simulink model "walkingRobotRL3D"  (R2020b)
settings: Solver=ode23t  StartTime=0.0  StopTime=Tf  RelTol=1e-2  EnableMultiTasking=on
PreLoadFcn:
  | robotParametersRL
undefined symbols (not defined in the file): agent, ankleD_pitch_jointMAX, ankleD_pitch_jointMIN, ankleD_roll_jointMAX, ankleD_roll_jointMIN, ankleI_pitch_jointMAX, ankleI_pitch_jointMIN, ankleI_roll_jointMAX, ankleI_roll_jointMIN, getSampleTime, height_plane, hipD_pitch_jointMAX, hipD_pitch_jointMIN, hipD_roll_jointMAX, hipD_roll_jointMIN, hipI_pitch_jointMAX, hipI_pitch_jointMIN, hipI_roll_jointMAX, hipI_roll_jointMIN, init_angs_L, init_angs_R, init_height, joint_damping, joint_limit_damping, joint_limit_stiffness, joint_stiffness, kneeD_jointMAX, kneeD_jointMIN, kneeI_jointMAX, kneeI_jointMIN, lower_leg_I0, lower_leg_length, lower_leg_mass, lower_leg_x, lower_leg_y, muscle_nominal_length, p10_ankleD_roll, plane_x, plane_y, regulator_type, tau, Tf, torso_height, torso_length, torso_offset_x, torso_offset_z, torso_width, torso_x, torso_y, torso_z, Ts, upper_leg_I0, upper_leg_length, upper_leg_mass, upper_leg_x, upper_leg_y, v10_ankleD_pitch, v10_ankleD_roll, v10_ankleI_pitch, v10_ankleI_roll ... (+41)
libraries: sm_lib x222, simulink x183, nesl_utility x130, walkingRobotUtils x69, rllib x2
(part 4 of 24)

== system walkingRobotRL3D/Calculate Reward3/Check correct behaviour of the muscles ==
  actions : Inport
  Add : Sum  Inputs=++++++++++
  Demux : Demux  Outputs=20
  Subsystem : Subsystem
  Subsystem1 : Subsystem
  Subsystem2 : Subsystem
  Subsystem3 : Subsystem
  Subsystem4 : Subsystem
  Subsystem5 : Subsystem
  Subsystem6 : Subsystem
  Subsystem7 : Subsystem
  Subsystem8 : Subsystem
  Subsystem9 : Subsystem
  Muscles checked : Outport
  wires:
  actions/1 -> Demux/1
  Demux/1 -> Subsystem/1(In1)
  Demux/2 -> Subsystem/2(In2)
  Subsystem/1(Out1) -> Add/1
  Demux/3 -> Subsystem1/1(In1)
  Demux/4 -> Subsystem1/2(In2)
  Subsystem1/1(Out1) -> Add/2
  Demux/7 -> Subsystem3/1(In1)
  Demux/8 -> Subsystem3/2(In2)
  Demux/9 -> Subsystem4/1(In1)
  Demux/10 -> Subsystem4/2(In2)
  Demux/11 -> Subsystem5/1(In1)
  Demux/12 -> Subsystem5/2(In2)
  Demux/13 -> Subsystem6/1(In1)
  Demux/14 -> Subsystem6/2(In2)
  Demux/17 -> Subsystem7/1(In1)
  Demux/18 -> Subsystem7/2(In2)
  Demux/19 -> Subsystem8/1(In1)
  Demux/20 -> Subsystem8/2(In2)
  Demux/5 -> Subsystem2/1(In1)
  Demux/6 -> Subsystem2/2(In2)
  Subsystem2/1(Out1) -> Add/3
  Subsystem3/1(Out1) -> Add/4
  Subsystem4/1(Out1) -> Add/5
  Subsystem5/1(Out1) -> Add/6
  Subsystem6/1(Out1) -> Add/7
  Subsystem9/1(Out1) -> Add/8
  Subsystem7/1(Out1) -> Add/9
  Subsystem8/1(Out1) -> Add/10
  Add/1 -> Muscles checked/1
  Demux/15 -> Subsystem9/1(In1)
  Demux/16 -> Subsystem9/2(In2)

== system walkingRobotRL3D/Calculate Reward3/Subsystem ==
  In1 : Inport
  Add{3..12} (10 alike) : Sum  Inputs=--
  Demux : Demux  Outputs=20
  use reward : Outport
  used reward1 : Outport  Port=2
  used reward2 : Outport  Port=3
  used reward3 : Outport  Port=4
  used reward4 : Outport  Port=5
  used reward5 : Outport  Port=6
  used reward6 : Outport  Port=7
  used reward7 : Outport  Port=8
  used reward8 : Outport  Port=9
  used reward9 : Outport  Port=10
  wires:
  Demux/10 -> Add7/2
  Demux/16 -> Add10/2
  Add5/1 -> used reward2/1  "kneeD"
  Demux/5 -> Add5/1
  Demux/19 -> Add12/1
  Demux/15 -> Add10/1
  Demux/11 -> Add8/1
  Demux/12 -> Add8/2
  Demux/2 -> Add3/2
  Demux/14 -> Add9/2
  Demux/3 -> Add4/1
  Add9/1 -> used reward6/1  "ankleI_pitch"
  Demux/1 -> Add3/1
  Demux/8 -> Add6/2
  Demux/20 -> Add12/2
  Demux/9 -> Add7/1
  Demux/4 -> Add4/2
  Demux/13 -> Add9/1
  Demux/7 -> Add6/1
  Add3/1 -> use reward/1  "ankleD_roll"
  Demux/6 -> Add5/2
  Demux/18 -> Add11/2
  Demux/17 -> Add11/1
  Add8/1 -> used reward5/1  "ankleI_roll"
  In1/1 -> Demux/1
  Add7/1 -> used reward4/1  "hipD_pitch"
  Add11/1 -> used reward8/1  "hipI_roll"
  Add10/1 -> used reward7/1  "kneeI"
  Add12/1 -> used reward9/1  "hipI_pitch"
  Add4/1 -> used reward1/1  "ankleD_pitch"
  Add6/1 -> used reward3/1  "hipD_roll"

== system walkingRobotRL3D/Calculate Reward3/Subsystem1 ==
  In1 : Inport
  Add : Sum  Inputs=++++++++++
  Add{4..13} (10 alike) : Sum  Inputs=+-
  Demux : Demux  Outputs=20
  Gain : Gain  Gain=1/10
  Square{,1..9} (10 alike) : Math  Operator=square  SaturateOnIntegerOverflow=on
  error to maximize : Outport
  wires:
  Demux/12 -> Add9/2
  Demux/2 -> Add4/2
  Demux/3 -> Add5/1
  Demux/9 -> Add8/1
  Demux/20 -> Add12/2
  Add10/1 -> Square7/1  "kneeI"
  Demux/17 -> Add11/1
  Demux/7 -> Add7/1
  Demux/14 -> Add13/2
  Demux/18 -> Add11/2
  Demux/4 -> Add5/2
  Demux/6 -> Add6/2
  Add9/1 -> Square5/1  "ankleI_roll"
  Demux/1 -> Add4/1
  Add12/1 -> Square9/1  "hipI_pitch"
  Demux/11 -> Add9/1
  Demux/8 -> Add7/2
  Add13/1 -> Square6/1  "ankleI_pitch"
  Demux/13 -> Add13/1
  Add11/1 -> Square8/1  "hipI_roll"
  Demux/19 -> Add12/1
  Demux/15 -> Add10/1
  Add4/1 -> Square/1  "ankleD_roll"
  Demux/10 -> Add8/2
  Demux/5 -> Add6/1
  Add8/1 -> Square4/1  "hipD_pitch"
  Demux/16 -> Add10/2
  Add7/1 -> Square3/1  "hipD_roll"
  Add6/1 -> Square2/1  "kneeD"
  In1/1 -> Demux/1
  Add5/1 -> Square1/1  "ankleD_pitch"
  Square1/1 -> Add/2
  Square2/1 -> Add/3
  Square3/1 -> Add/4
  Square4/1 -> Add/5
  Square5/1 -> Add/6
  Square6/1 -> Add/7
  Square7/1 -> Add/8
  Square8/1 -> Add/9
  Add/1 -> Gain/1
  Gain/1 -> error to maximize/1
  Square/1 -> Add/1
  Square9/1 -> Add/10

== system walkingRobotRL3D/Check if Done22/Check correct behaviour of the muscles ==
  actions : Inport
  Add : Sum  Inputs=++++++++++
  Demux : Demux  Outputs=20
  Subsystem : Subsystem
  Subsystem1 : Subsystem
  Subsystem2 : Subsystem
  Subsystem3 : Subsystem
  Subsystem4 : Subsystem
  Subsystem5 : Subsystem
  Subsystem6 : Subsystem
  Subsystem7 : Subsystem
  Subsystem8 : Subsystem
  Subsystem9 : Subsystem
  Muscles checked : Outport
  wires:
  actions/1 -> Demux/1
  Demux/1 -> Subsystem/1(In1)
  Demux/2 -> Subsystem/2(In2)
  Subsystem/1(Out1) -> Add/1
  Demux/3 -> Subsystem1/1(In1)
  Demux/4 -> Subsystem1/2(In2)
  Subsystem1/1(Out1) -> Add/2
  Demux/7 -> Subsystem3/1(In1)
  Demux/8 -> Subsystem3/2(In2)
  Demux/9 -> Subsystem4/1(In1)
  Demux/10 -> Subsystem4/2(In2)
  Demux/11 -> Subsystem5/1(In1)
  Demux/12 -> Subsystem5/2(In2)
  Demux/13 -> Subsystem6/1(In1)
  Demux/14 -> Subsystem6/2(In2)
  Demux/17 -> Subsystem7/1(In1)
  Demux/18 -> Subsystem7/2(In2)
  Demux/19 -> Subsystem8/1(In1)
  Demux/20 -> Subsystem8/2(In2)
  Demux/5 -> Subsystem2/1(In1)
  Demux/6 -> Subsystem2/2(In2)
  Subsystem2/1(Out1) -> Add/3
  Subsystem3/1(Out1) -> Add/4
  Subsystem4/1(Out1) -> Add/5
  Subsystem5/1(Out1) -> Add/6
  Subsystem6/1(Out1) -> Add/7
  Subsystem9/1(Out1) -> Add/8
  Subsystem7/1(Out1) -> Add/9
  Subsystem8/1(Out1) -> Add/10
  Add/1 -> Muscles checked/1
  Demux/15 -> Subsystem9/1(In1)
  Demux/16 -> Subsystem9/2(In2)

== system walkingRobotRL3D/Check if Done3/Check correct behaviour of the muscles ==
  actions : Inport
  Add : Sum  Inputs=++++++++++
  Demux : Demux  Outputs=20
  Subsystem : Subsystem
  Subsystem1 : Subsystem
  Subsystem2 : Subsystem
  Subsystem3 : Subsystem
  Subsystem4 : Subsystem
  Subsystem5 : Subsystem
  Subsystem6 : Subsystem
  Subsystem7 : Subsystem
  Subsystem8 : Subsystem
  Subsystem9 : Subsystem
  Muscles checked : Outport
  wires:
  actions/1 -> Demux/1
  Demux/1 -> Subsystem/1(In1)
  Demux/2 -> Subsystem/2(In2)
  Subsystem/1(Out1) -> Add/1
  Demux/3 -> Subsystem1/1(In1)
  Demux/4 -> Subsystem1/2(In2)
  Subsystem1/1(Out1) -> Add/2
  Demux/7 -> Subsystem3/1(In1)
  Demux/8 -> Subsystem3/2(In2)
  Demux/9 -> Subsystem4/1(In1)
  Demux/10 -> Subsystem4/2(In2)
  Demux/11 -> Subsystem5/1(In1)
  Demux/12 -> Subsystem5/2(In2)
  Demux/13 -> Subsystem6/1(In1)
  Demux/14 -> Subsystem6/2(In2)
  Demux/17 -> Subsystem7/1(In1)
  Demux/18 -> Subsystem7/2(In2)
  Demux/19 -> Subsystem8/1(In1)
  Demux/20 -> Subsystem8/2(In2)
  Demux/5 -> Subsystem2/1(In1)
  Demux/6 -> Subsystem2/2(In2)
  Subsystem2/1(Out1) -> Add/3
  Subsystem3/1(Out1) -> Add/4
  Subsystem4/1(Out1) -> Add/5
  Subsystem5/1(Out1) -> Add/6
  Subsystem6/1(Out1) -> Add/7
  Subsystem9/1(Out1) -> Add/8
  Subsystem7/1(Out1) -> Add/9
  Subsystem8/1(Out1) -> Add/10
  Add/1 -> Muscles checked/1
  Demux/15 -> Subsystem9/1(In1)
  Demux/16 -> Subsystem9/2(In2)

== system walkingRobotRL3D/RL Agent3/accumulate_reward ==
  reward : Inport
  Constant : Constant
  Rate Transition : RateTransition  OutPortSampleTime=getSampleTime(Agent)
  Unit Delay : UnitDelay  SampleTime=-1  HasFrameUpgradeWarning=on
  cumsum : Subsystem
  cumulative_reward : Outport  VectorParamsAs1DForOutWhenUnconnected=off
  wires:
  Rate Transition/1 -> cumsum/1(rwd)
  reward/1 -> Rate Transition/1
  Constant/1 -> Unit Delay/1
  Unit Delay/1 -> cumsum/Enable
  cumsum/1(cumulative_rwd) -> cumulative_reward/1

== system walkingRobotRL3D/RL Agent33/accumulate_reward ==
  reward : Inport
  Constant : Constant
  Rate Transition : RateTransition  OutPortSampleTime=getSampleTime(Agent)
  Unit Delay : UnitDelay  SampleTime=-1  HasFrameUpgradeWarning=on
  cumsum : Subsystem
  cumulative_reward : Outport  VectorParamsAs1DForOutWhenUnconnected=off
  wires:
  Rate Transition/1 -> cumsum/1(rwd)
  reward/1 -> Rate Transition/1
  Constant/1 -> Unit Delay/1
  Unit Delay/1 -> cumsum/Enable
  cumsum/1(cumulative_rwd) -> cumulative_reward/1

== system walkingRobotRL3D/Walking Robot/DYNAMIC MODEL OF PAM FOR LEFT LEG ==
  In1 : Inport
  In2 : Inport  Port=2
  In3 : Inport  Port=3
  In4 : Inport  Port=4
  In5 : Inport  Port=5
  In6 : Inport  Port=6
  In7 : Inport  Port=7
  In8 : Inport  Port=8
  In9 : Inport  Port=9
  In10 : Inport  Port=10
  Dynamic Model Antagonisitic PAM1 : Subsystem
  Dynamic Model Antagonisitic PAM2 : Subsystem
  Dynamic Model Antagonisitic PAM3 : Subsystem
  Dynamic Model Antagonisitic PAM4 : Subsystem
  Dynamic Model Antagonisitic PAM5 : Subsystem
  F-->Torque1 : MATLAB Function  TreatAsAtomicUnit=on
  F-->Torque2 : MATLAB Function  TreatAsAtomicUnit=on
  F-->Torque3 : MATLAB Function  TreatAsAtomicUnit=on
  F-->Torque4 : MATLAB Function  TreatAsAtomicUnit=on
  F-->Torque5 : MATLAB Function  TreatAsAtomicUnit=on
  Mux : Mux  Inputs=5
  Out1 : Outport
  wires:
  Dynamic Model Antagonisitic PAM5/1(F1) -> F-->Torque5/1(R1)
  Dynamic Model Antagonisitic PAM1/1(F1) -> F-->Torque1/1(R1)
  Dynamic Model Antagonisitic PAM3/2(F2) -> F-->Torque3/2(R2)
  Dynamic Model Antagonisitic PAM5/2(F2) -> F-->Torque5/2(R2)
  F-->Torque3/1(torque) -> Mux/1
  F-->Torque5/1(torque) -> Mux/5
  In7/1 -> Dynamic Model Antagonisitic PAM4/1(V1)
  In1/1 -> Dynamic Model Antagonisitic PAM3/1(V1)
  In3/1 -> Dynamic Model Antagonisitic PAM1/1(V1)
  F-->Torque1/1(torque) -> Mux/2
  Dynamic Model Antagonisitic PAM2/2(F2) -> F-->Torque2/2(R2)
  In8/1 -> Dynamic Model Antagonisitic PAM4/2(V2)
  In4/1 -> Dynamic Model Antagonisitic PAM1/2(V2)
  Dynamic Model Antagonisitic PAM2/1(F1) -> F-->Torque2/1(R1)
  F-->Torque4/1(torque) -> Mux/4
  Dynamic Model Antagonisitic PAM3/1(F1) -> F-->Torque3/1(R1)
  F-->Torque2/1(torque) -> Mux/3
  Dynamic Model Antagonisitic PAM4/2(F2) -> F-->Torque4/2(R2)
  Dynamic Model Antagonisitic PAM4/1(F1) -> F-->Torque4/1(R1)
  Dynamic Model Antagonisitic PAM1/2(F2) -> F-->Torque1/2(R2)
  Mux/1 -> Out1/1
  In9/1 -> Dynamic Model Antagonisitic PAM5/1(V1)
  In6/1 -> Dynamic Model Antagonisitic PAM2/2(V2)
  In5/1 -> Dynamic Model Antagonisitic PAM2/1(V1)
  In10/1 -> Dynamic Model Antagonisitic PAM5/2(V2)
  In2/1 -> Dynamic Model Antagonisitic PAM3/2(V2)

== system walkingRobotRL3D/Walking Robot/DYNAMIC MODEL OF PAM FOR RIGHT LEG ==
  In1 : Inport
  In2 : Inport  Port=2
  In3 : Inport  Port=3
  In4 : Inport  Port=4
  In5 : Inport  Port=5
  In6 : Inport  Port=6
  In7 : Inport  Port=7
  In8 : Inport  Port=8
  In9 : Inport  Port=9
  In10 : Inport  Port=10
  Dynamic Model Antagonisitic PAM1 : Subsystem
  Dynamic Model Antagonisitic PAM2 : Subsystem
  Dynamic Model Antagonisitic PAM3 : Subsystem
  Dynamic Model Antagonisitic PAM4 : Subsystem
  Dynamic Model Antagonisitic PAM5 : Subsystem
  F-->Torque1 : MATLAB Function  TreatAsAtomicUnit=on
  F-->Torque2 : MATLAB Function  TreatAsAtomicUnit=on
  F-->Torque3 : MATLAB Function  TreatAsAtomicUnit=on
  F-->Torque4 : MATLAB Function  TreatAsAtomicUnit=on
  F-->Torque5 : MATLAB Function  TreatAsAtomicUnit=on
  Mux : Mux  Inputs=5
  Out1 : Outport
  wires:
  Dynamic Model Antagonisitic PAM5/1(F1) -> F-->Torque5/1(R1)
  Dynamic Model Antagonisitic PAM1/1(F1) -> F-->Torque1/1(R1)
  Dynamic Model Antagonisitic PAM3/2(F2) -> F-->Torque3/2(R2)
  Dynamic Model Antagonisitic PAM5/2(F2) -> F-->Torque5/2(R2)
  F-->Torque3/1(torque) -> Mux/1
  F-->Torque5/1(torque) -> Mux/5
  In7/1 -> Dynamic Model Antagonisitic PAM4/1(V1)
  In1/1 -> Dynamic Model Antagonisitic PAM3/1(V1)
  In3/1 -> Dynamic Model Antagonisitic PAM1/1(V1)
  F-->Torque1/1(torque) -> Mux/2
  Dynamic Model Antagonisitic PAM2/2(F2) -> F-->Torque2/2(R2)
  In8/1 -> Dynamic Model Antagonisitic PAM4/2(V2)
  In4/1 -> Dynamic Model Antagonisitic PAM1/2(V2)
  Dynamic Model Antagonisitic PAM2/1(F1) -> F-->Torque2/1(R1)
  F-->Torque4/1(torque) -> Mux/4
  Dynamic Model Antagonisitic PAM3/1(F1) -> F-->Torque3/1(R1)
  F-->Torque2/1(torque) -> Mux/3
  Dynamic Model Antagonisitic PAM4/2(F2) -> F-->Torque4/2(R2)
  Dynamic Model Antagonisitic PAM4/1(F1) -> F-->Torque4/1(R1)
  Dynamic Model Antagonisitic PAM1/2(F2) -> F-->Torque1/2(R2)
  Mux/1 -> Out1/1
  In9/1 -> Dynamic Model Antagonisitic PAM5/1(V1)
  In6/1 -> Dynamic Model Antagonisitic PAM2/2(V2)
  In5/1 -> Dynamic Model Antagonisitic PAM2/1(V1)
  In10/1 -> Dynamic Model Antagonisitic PAM5/2(V2)
  In2/1 -> Dynamic Model Antagonisitic PAM3/2(V2)

== system walkingRobotRL3D/Walking Robot/Robot Leg L ==
  torques : Inport
  Ankle Pitch to Roll : sm_lib/Frames and Transforms/Rigid Transform  TranslationMethod=None  TranslationStandardOffset=0  TranslationLengthUnit=m  TranslationStandardAxis=+Z  TranslationCartesianOffset=[0 0 0]  TranslationROffset=0  TranslationROffsetUnits=m  TranslationZOffset=0  TranslationZOffsetUnits=m  TranslationThetaOffset=0  TranslationThetaOffsetUnits=deg  RotationMethod=StandardAxis  RotationAngleUnits=deg  RotationStandardAxis=+Y  RotationAngle=90  RotationArbitraryAxis=[0 0 1]  FollAlignAxisA=+X  BaseAlignAxisA=+Y  FollAlignAxisB=+Y  BaseAlignAxisB=+Z  RotationSequenceAxes=FollowerAxes  RotationSequence=XYX  RotationSequenceAngles=[0 0 0]  RotationSequenceAnglesUnits=deg  RotationMatrix=[1 0 0; 0 1 0; 0 0 1]
  Ankle Roll to Pitch : sm_lib/Frames and Transforms/Rigid Transform  TranslationMethod=None  TranslationStandardOffset=0  TranslationLengthUnit=m  TranslationStandardAxis=+Z  TranslationCartesianOffset=[0 0 0]  TranslationROffset=0  TranslationROffsetUnits=m  TranslationZOffset=0  TranslationZOffsetUnits=m  TranslationThetaOffset=0  TranslationThetaOffsetUnits=deg  RotationMethod=StandardAxis  RotationAngleUnits=deg  RotationStandardAxis=+Y  RotationAngle=-90  RotationArbitraryAxis=[0 0 1]  FollAlignAxisA=+X  BaseAlignAxisA=+Y  FollAlignAxisB=+Y  BaseAlignAxisB=+Z  RotationSequenceAxes=FollowerAxes  RotationSequence=XYX  RotationSequenceAngles=[0 0 0]  RotationSequenceAnglesUnits=deg  RotationMatrix=[1 0 0; 0 1 0; 0 0 1]
  Ankle Pitch Joint : walkingRobotUtils/Leg Joint with Limits  VariantControl=actuatorType == 2  k=joint_stiffness  d=joint_damping  initAngle=init_angs_L(2)  eqAngle=0  upperLimit=pi/4  lowerLimit=-pi/4  jointLimitStiffness=joint_limit_stiffness  jointLimitDamping=joint_limit_damping
  Ankle Roll Joint : walkingRobotUtils/Leg Joint with Limits  VariantControl=actuatorType == 2  k=joint_stiffness  d=joint_damping  initAngle=init_angs_L(1)  eqAngle=0  upperLimit=pi/16  lowerLimit=-pi/16  jointLimitStiffness=joint_limit_stiffness  jointLimitDamping=joint_limit_damping
  Ankle to Lower Leg : sm_lib/Frames and Transforms/Rigid Transform  TranslationMethod=Cartesian  TranslationStandardOffset=0  TranslationLengthUnit=cm  TranslationStandardAxis=+Z  TranslationCartesianOffset=[0 lower_leg_length/2 0]  TranslationROffset=0  TranslationROffsetUnits=m  TranslationZOffset=0  TranslationZOffsetUnits=m  TranslationThetaOffset=0  TranslationThetaOffsetUnits=deg  RotationMethod=StandardAxis  RotationAngleUnits=deg  RotationStandardAxis=+X  RotationAngle=-90  RotationArbitraryAxis=[0 0 1]  FollAlignAxisA=+X  BaseAlignAxisA=+Y  FollAlignAxisB=+Y  BaseAlignAxisB=+Z  RotationSequenceAxes=FollowerAxes  RotationSequence=XYX  RotationSequenceAngles=[0 0 0]  RotationSequenceAnglesUnits=deg  RotationMatrix=[1 0 0; 0 1 0; 0 0 1]
  Demux : Demux  Outputs=5
  Foot Offset : sm_lib/Frames and Transforms/Rigid Transform  TranslationMethod=Cartesian  TranslationStandardOffset=0  TranslationLengthUnit=cm  TranslationStandardAxis=+Z  TranslationCartesianOffset=foot_offset  TranslationROffset=0  TranslationROffsetUnits=m  TranslationZOffset=0  TranslationZOffsetUnits=m  TranslationThetaOffset=0  TranslationThetaOffsetUnits=deg  RotationMethod=None  RotationAngleUnits=deg  RotationStandardAxis=+X  RotationAngle=-90  RotationArbitraryAxis=[0 0 1]  FollAlignAxisA=+X  BaseAlignAxisA=+Y  FollAlignAxisB=+Y  BaseAlignAxisB=+Z  RotationSequenceAxes=FollowerAxes  RotationSequence=XYX  RotationSequenceAngles=[0 0 0]  RotationSequenceAnglesUnits=deg  RotationMatrix=[1 0 0; 0 1 0; 0 0 1]
  Foot and Contact : walkingRobotUtils/Walking Robot (Control Design)/Robot Leg R/Foot and Contact  SystemSampleTime=-1  VariantActivationTime=update diagram  Latency=0  AutoFrameSizeCalculation=off
      link override Foot: GraphicDiffuseColor=[1.0 0.0 0.0]
  Hip Pitch to Roll : sm_lib/Frames and Transforms/Rigid Transform  TranslationMethod=None  TranslationStandardOffset=0  TranslationLengthUnit=m  TranslationStandardAxis=+Z  TranslationCartesianOffset=[0 0 0]  TranslationROffset=0  TranslationROffsetUnits=m  TranslationZOffset=0  TranslationZOffsetUnits=m  TranslationThetaOffset=0  TranslationThetaOffsetUnits=deg  RotationMethod=StandardAxis  RotationAngleUnits=deg  RotationStandardAxis=+Y  RotationAngle=90  RotationArbitraryAxis=[0 0 1]  FollAlignAxisA=+X  BaseAlignAxisA=+Y  FollAlignAxisB=+Y  BaseAlignAxisB=+Z  RotationSequenceAxes=FollowerAxes  RotationSequence=XYX  RotationSequenceAngles=[0 0 0]  RotationSequenceAnglesUnits=deg  RotationMatrix=[1 0 0; 0 1 0; 0 0 1]
  Hip Roll to Pitch : sm_lib/Frames and Transforms/Rigid Transform  TranslationMethod=None  TranslationStandardOffset=0  TranslationLengthUnit=m  TranslationStandardAxis=+Z  TranslationCartesianOffset=[0 0 0]  TranslationROffset=0  TranslationROffsetUnits=m  TranslationZOffset=0  TranslationZOffsetUnits=m  TranslationThetaOffset=0  TranslationThetaOffsetUnits=deg  RotationMethod=StandardAxis  RotationAngleUnits=deg  RotationStandardAxis=+Y  RotationAngle=-90  RotationArbitraryAxis=[0 0 1]  FollAlignAxisA=+X  BaseAlignAxisA=+Y  FollAlignAxisB=+Y  BaseAlignAxisB=+Z  RotationSequenceAxes=FollowerAxes  RotationSequence=XYX  RotationSequenceAngles=[0 0 0]  RotationSequenceAnglesUnits=deg  RotationMatrix=[1 0 0; 0 1 0; 0 0 1]
  Hip Pitch Joint : walkingRobotUtils/Leg Joint with Limits  VariantControl=actuatorType == 2  k=joint_stiffness  d=joint_damping  initAngle=init_angs_L(5)  eqAngle=0  upperLimit=pi/4  lowerLimit=-pi/4  jointLimitStiffness=joint_limit_stiffness  jointLimitDamping=joint_limit_damping
  Hip Roll Joint : walkingRobotUtils/Leg Joint with Limits  VariantControl=actuatorType == 2  k=joint_stiffness  d=joint_damping  initAngle=init_angs_L(4)  eqAngle=0  upperLimit=0  lowerLimit=-pi/16  jointLimitStiffness=joint_limit_stiffness  jointLimitDamping=joint_limit_damping
  Hip to World Coords : sm_lib/Frames and Transforms/Rigid Transform  TranslationMethod=None  TranslationStandardOffset=0  TranslationLengthUnit=cm  TranslationStandardAxis=+Z  TranslationCartesianOffset=[0 0 upper_leg_length/2]  TranslationROffset=0  TranslationROffsetUnits=m  TranslationZOffset=0  TranslationZOffsetUnits=m  TranslationThetaOffset=0  TranslationThetaOffsetUnits=deg  RotationMethod=StandardAxis  RotationAngleUnits=deg  RotationStandardAxis=+X  RotationAngle=-90  RotationArbitraryAxis=[0 0 1]  FollAlignAxisA=+X  BaseAlignAxisA=+Y  FollAlignAxisB=+Y  BaseAlignAxisB=+Z  RotationSequenceAxes=FollowerAxes  RotationSequence=XYX  RotationSequenceAngles=[0 0 0]  RotationSequenceAnglesUnits=deg  RotationMatrix=[1 0 0; 0 1 0; 0 0 1]
  Knee Joint : walkingRobotUtils/Leg Joint with Limits  VariantControl=actuatorType == 2  k=joint_stiffness  d=joint_damping  initAngle=init_angs_L(3)  eqAngle=0  upperLimit=pi/2  lowerLimit=0  jointLimitStiffness=joint_limit_stiffness  jointLimitDamping=joint_limit_damping
  Knee to Upper Leg : sm_lib/Frames and Transforms/Rigid Transform  TranslationMethod=Cartesian  TranslationStandardOffset=0  TranslationLengthUnit=cm  TranslationStandardAxis=+Z  TranslationCartesianOffset=[0 upper_leg_length/2 0]  TranslationROffset=0  TranslationROffsetUnits=m  TranslationZOffset=0  TranslationZOffsetUnits=m  TranslationThetaOffset=0  TranslationThetaOffsetUnits=deg  RotationMethod=StandardAxis  RotationAngleUnits=deg  RotationStandardAxis=+X  RotationAngle=-90  RotationArbitraryAxis=[0 0 1]  FollAlignAxisA=+X  BaseAlignAxisA=+Y  FollAlignAxisB=+Y  BaseAlignAxisB=+Z  RotationSequenceAxes=FollowerAxes  RotationSequence=XYX  RotationSequenceAngles=[0 0 0]  RotationSequenceAnglesUnits=deg  RotationMatrix=[1 0 0; 0 1 0; 0 0 1]
  Lower Leg : sm_lib/Body Elements/Cylindrical Solid  GraphicAmbientColor=[0.15 0.15 0.15 1.0]  BasedOnType=Density  CenterOfMass=[0 0 0]  CenterOfMassUnits=m  GraphicDiffuseColor=[0.0 0.8 0.0]  CylinderLength=lower_leg_length  CylinderLengthUnits=cm  CylinderRadius=leg_radius  CylinderRadiusUnits=cm  Density=density  DensityUnits=kg/m^3  DoExposeReferenceFrame=on  GraphicEmissiveColor=[0.0 0.0 0.0 1.0]  ExportEntireGeometry=off  SerializedFrames=<Frames/>  MarkerShape=Sphere  MarkerSize=10  GraphicType=FromGeometry  InertiaType=CalculateFromGeometry  Mass=1  MassUnits=kg  MomentsOfInertia=[1 1 1]  MomentsOfInertiaUnits=kg*m^2  GraphicOpacity=1.0  ProductsOfInertia=[1 1 1]  ProductsOfInertiaUnits=kg*m^2  GraphicShininess=75  GraphicSpecularColor=[0.5 0.5 0.5 1.0]  GraphicVisPropType=SimpleVisualProperties
  Lower Leg to Knee : sm_lib/Frames and Transforms/Rigid Transform  TranslationMethod=Cartesian  TranslationStandardOffset=0  TranslationLengthUnit=cm  TranslationStandardAxis=+Z  TranslationCartesianOffset=[0 0 lower_leg_length/2]  TranslationROffset=0  TranslationROffsetUnits=m  TranslationZOffset=0  TranslationZOffsetUnits=m  TranslationThetaOffset=0  TranslationThetaOffsetUnits=deg  RotationMethod=StandardAxis  RotationAngleUnits=deg  RotationStandardAxis=+X  RotationAngle=90  RotationArbitraryAxis=[0 0 1]  FollAlignAxisA=+X  BaseAlignAxisA=+Y  FollAlignAxisB=+Y  BaseAlignAxisB=+Z  RotationSequenceAxes=FollowerAxes  RotationSequence=XYX  RotationSequenceAngles=[0 0 0]  RotationSequenceAnglesUnits=deg  RotationMatrix=[1 0 0; 0 1 0; 0 0 1]
  Package Measurements 3D : walkingRobotUtils/Package Measurements 3D  SystemSampleTime=-1  VariantActivationTime=update diagram  Latency=0  AutoFrameSizeCalculation=off
  Upper Leg : sm_lib/Body Elements/Cylindrical Solid  GraphicAmbientColor=[0.15 0.15 0.15 1.0]  BasedOnType=Density  CenterOfMass=[0 0 0]  CenterOfMassUnits=m  GraphicDiffuseColor=[0.0 0.0 1.0]  CylinderLength=upper_leg_length  CylinderLengthUnits=cm  CylinderRadius=leg_radius  CylinderRadiusUnits=cm  Density=density  DensityUnits=kg/m^3  DoExposeReferenceFrame=on  GraphicEmissiveColor=[0.0 0.0 0.0 1.0]  ExportEntireGeometry=off  SerializedFrames=<Frames/>  MarkerShape=Sphere  MarkerSize=10  GraphicType=FromGeometry  InertiaType=CalculateFromGeometry  Mass=1  MassUnits=kg  MomentsOfInertia=[1 1 1]  MomentsOfInertiaUnits=kg*m^2  GraphicOpacity=1.0  ProductsOfInertia=[1 1 1]  ProductsOfInertiaUnits=kg*m^2  GraphicShininess=75  GraphicSpecularColor=[0.5 0.5 0.5 1.0]  GraphicVisPropType=SimpleVisualProperties
  Upper Leg to Hip : sm_lib/Frames and Transforms/Rigid Transform  TranslationMethod=Cartesian  TranslationStandardOffset=0  TranslationLengthUnit=cm  TranslationStandardAxis=+Z  TranslationCartesianOffset=[0 0 upper_leg_length/2]  TranslationROffset=0  TranslationROffsetUnits=m  TranslationZOffset=0  TranslationZOffsetUnits=m  TranslationThetaOffset=0  TranslationThetaOffsetUnits=deg  RotationMethod=StandardAxis  RotationAngleUnits=deg  RotationStandardAxis=+X  RotationAngle=90  RotationArbitraryAxis=[0 0 1]  FollAlignAxisA=+X  BaseAlignAxisA=+Y  FollAlignAxisB=+Y  BaseAlignAxisB=+Z  RotationSequenceAxes=FollowerAxes  RotationSequence=XYX  RotationSequenceAngles=[0 0 0]  RotationSequenceAnglesUnits=deg  RotationMatrix=[1 0 0; 0 1 0; 0 0 1]
  G : PMIOPort  Side=Right
  H : PMIOPort  Port=2  Side=Right
  meas : Outport  VectorParamsAs1DForOutWhenUnconnected=off
  wires:
  Ankle Roll Joint/1 -> Package Measurements 3D/3
  Hip Roll Joint/1 -> Package Measurements 3D/6
  Demux/5 -> Hip Pitch Joint/1
  Demux/4 -> Hip Roll Joint/1
  Demux/3 -> Knee Joint/1
  Demux/2 -> Ankle Pitch Joint/1
  Demux/1 -> Ankle Roll Joint/1
  torques/1 -> Demux/1
  Ankle Pitch Joint/1 -> Package Measurements 3D/4
  Package Measurements 3D/1 -> meas/1
  Hip Pitch Joint/1 -> Package Measurements 3D/7
  Knee Joint/1 -> Package Measurements 3D/5
  Foot and Contact/2 -> Package Measurements 3D/2
  Foot and Contact/1 -> Package Measurements 3D/1
  connections:
  Hip Roll to Pitch/RConn1 -- Hip Pitch Joint/LConn1
  Upper Leg to Hip/RConn1 -- Hip Pitch to Roll/LConn1
  Ankle Pitch Joint/LConn1 -- Ankle Roll to Pitch/RConn1
  Foot Offset/RConn1 -- Ankle Pitch to Roll/LConn1
  Hip Roll Joint/RConn1 -- Hip Roll to Pitch/LConn1
  Hip Roll Joint/LConn1 -- Hip Pitch to Roll/RConn1
  Hip Pitch Joint/RConn1 -- Hip to World Coords/LConn1
  Ankle Pitch Joint/RConn1 -- Ankle to Lower Leg/LConn1
  Ankle Roll Joint/RConn1 -- Ankle Roll to Pitch/LConn1
  Ankle Roll Joint/LConn1 -- Ankle Pitch to Roll/RConn1
  Knee Joint/RConn1 -- Knee to Upper Leg/LConn1
  G/RConn1 -- Foot and Contact/LConn1
  Ankle to Lower Leg/RConn1 -- Lower Leg/RConn1 -- Lower Leg to Knee/LConn1
  Upper Leg to Hip/LConn1 -- Upper Leg/RConn1 -- Knee to Upper Leg/RConn1
  Knee Joint/LConn1 -- Lower Leg to Knee/RConn1
  H/RConn1 -- Hip to World Coords/RConn1
  Foot and Contact/RConn1 -- Foot Offset/LConn1

== system walkingRobotRL3D/Walking Robot/Robot Leg R ==
  torques : Inport
  Ankle Pitch to Roll : sm_lib/Frames and Transforms/Rigid Transform  TranslationMethod=None  TranslationStandardOffset=0  TranslationLengthUnit=m  TranslationStandardAxis=+Z  TranslationCartesianOffset=[0 0 0]  TranslationROffset=0  TranslationROffsetUnits=m  TranslationZOffset=0  TranslationZOffsetUnits=m  TranslationThetaOffset=0  TranslationThetaOffsetUnits=deg  RotationMethod=StandardAxis  RotationAngleUnits=deg  RotationStandardAxis=+Y  RotationAngle=90  RotationArbitraryAxis=[0 0 1]  FollAlignAxisA=+X  BaseAlignAxisA=+Y  FollAlignAxisB=+Y  BaseAlignAxisB=+Z  RotationSequenceAxes=FollowerAxes  RotationSequence=XYX  RotationSequenceAngles=[0 0 0]  RotationSequenceAnglesUnits=deg  RotationMatrix=[1 0 0; 0 1 0; 0 0 1]
  Ankle Roll to Pitch : sm_lib/Frames and Transforms/Rigid Transform  TranslationMethod=None  TranslationStandardOffset=0  TranslationLengthUnit=m  TranslationStandardAxis=+Z  TranslationCartesianOffset=[0 0 0]  TranslationROffset=0  TranslationROffsetUnits=m  TranslationZOffset=0  TranslationZOffsetUnits=m  TranslationThetaOffset=0  TranslationThetaOffsetUnits=deg  RotationMethod=StandardAxis  RotationAngleUnits=deg  RotationStandardAxis=+Y  RotationAngle=-90  RotationArbitraryAxis=[0 0 1]  FollAlignAxisA=+X  BaseAlignAxisA=+Y  FollAlignAxisB=+Y  BaseAlignAxisB=+Z  RotationSequenceAxes=FollowerAxes  RotationSequence=XYX  RotationSequenceAngles=[0 0 0]  RotationSequenceAnglesUnits=deg  RotationMatrix=[1 0 0; 0 1 0; 0 0 1]
  Ankle Pitch Joint : walkingRobotUtils/Leg Joint with Limits  VariantControl=actuatorType == 2  k=joint_stiffness  d=joint_damping  initAngle=init_angs_R(2)  eqAngle=0  upperLimit=pi/4  lowerLimit=-pi/4  jointLimitStiffness=joint_limit_stiffness  jointLimitDamping=joint_limit_damping
  Ankle Roll Joint : walkingRobotUtils/Leg Joint with Limits  VariantControl=actuatorType == 2  k=joint_stiffness  d=joint_damping  initAngle=init_angs_R(1)  eqAngle=0  upperLimit=pi/16  lowerLimit=-pi/16  jointLimitStiffness=joint_limit_stiffness  jointLimitDamping=joint_limit_damping
  Ankle to Lower Leg : sm_lib/Frames and Transforms/Rigid Transform  TranslationMethod=Cartesian  TranslationStandardOffset=0  TranslationLengthUnit=cm  TranslationStandardAxis=+Z  TranslationCartesianOffset=[0 lower_leg_length/2 0]  TranslationROffset=0  TranslationROffsetUnits=m  TranslationZOffset=0  TranslationZOffsetUnits=m  TranslationThetaOffset=0  TranslationThetaOffsetUnits=deg  RotationMethod=StandardAxis  RotationAngleUnits=deg  RotationStandardAxis=+X  RotationAngle=-90  RotationArbitraryAxis=[0 0 1]  FollAlignAxisA=+X  BaseAlignAxisA=+Y  FollAlignAxisB=+Y  BaseAlignAxisB=+Z  RotationSequenceAxes=FollowerAxes  RotationSequence=XYX  RotationSequenceAngles=[0 0 0]  RotationSequenceAnglesUnits=deg  RotationMatrix=[1 0 0; 0 1 0; 0 0 1]
  Demux : Demux  Outputs=5
  Foot Offset : sm_lib/Frames and Transforms/Rigid Transform  TranslationMethod=Cartesian  TranslationStandardOffset=0  TranslationLengthUnit=cm  TranslationStandardAxis=+Z  TranslationCartesianOffset=foot_offset  TranslationROffset=0  TranslationROffsetUnits=m  TranslationZOffset=0  TranslationZOffsetUnits=m  TranslationThetaOffset=0  TranslationThetaOffsetUnits=deg  RotationMethod=None  RotationAngleUnits=deg  RotationStandardAxis=+X  RotationAngle=-90  RotationArbitraryAxis=[0 0 1]  FollAlignAxisA=+X  BaseAlignAxisA=+Y  FollAlignAxisB=+Y  BaseAlignAxisB=+Z  RotationSequenceAxes=FollowerAxes  RotationSequence=XYX  RotationSequenceAngles=[0 0 0]  RotationSequenceAnglesUnits=deg  RotationMatrix=[1 0 0; 0 1 0; 0 0 1]
  Foot and Contact : walkingRobotUtils/Walking Robot (Control Design)/Robot Leg R/Foot and Contact  SystemSampleTime=-1  VariantActivationTime=update diagram  Latency=0  AutoFrameSizeCalculation=off
      link override Foot: GraphicDiffuseColor=[1.0 0.0 0.0]
  Hip Pitch to Roll : sm_lib/Frames and Transforms/Rigid Transform  TranslationMethod=None  TranslationStandardOffset=0  TranslationLengthUnit=m  TranslationStandardAxis=+Z  TranslationCartesianOffset=[0 0 0]  TranslationROffset=0  TranslationROffsetUnits=m  TranslationZOffset=0  TranslationZOffsetUnits=m  TranslationThetaOffset=0  TranslationThetaOffsetUnits=deg  RotationMethod=StandardAxis  RotationAngleUnits=deg  RotationStandardAxis=+Y  RotationAngle=90  RotationArbitraryAxis=[0 0 1]  FollAlignAxisA=+X  BaseAlignAxisA=+Y  FollAlignAxisB=+Y  BaseAlignAxisB=+Z  RotationSequenceAxes=FollowerAxes  RotationSequence=XYX  RotationSequenceAngles=[0 0 0]  RotationSequenceAnglesUnits=deg  RotationMatrix=[1 0 0; 0 1 0; 0 0 1]
  Hip Roll to Pitch : sm_lib/Frames and Transforms/Rigid Transform  TranslationMethod=None  TranslationStandardOffset=0  TranslationLengthUnit=m  TranslationStandardAxis=+Z  TranslationCartesianOffset=[0 0 0]  TranslationROffset=0  TranslationROffsetUnits=m  TranslationZOffset=0  TranslationZOffsetUnits=m  TranslationThetaOffset=0  TranslationThetaOffsetUnits=deg  RotationMethod=StandardAxis  RotationAngleUnits=deg  RotationStandardAxis=+Y  RotationAngle=-90  RotationArbitraryAxis=[0 0 1]  FollAlignAxisA=+X  BaseAlignAxisA=+Y  FollAlignAxisB=+Y  BaseAlignAxisB=+Z  RotationSequenceAxes=FollowerAxes  RotationSequence=XYX  RotationSequenceAngles=[0 0 0]  RotationSequenceAnglesUnits=deg  RotationMatrix=[1 0 0; 0 1 0; 0 0 1]
  Hip Pitch Joint : walkingRobotUtils/Leg Joint with Limits  VariantControl=actuatorType == 2  k=joint_stiffness  d=joint_damping  initAngle=init_angs_R(5)  eqAngle=0  upperLimit=pi/4  lowerLimit=-pi/4  jointLimitStiffness=joint_limit_stiffness  jointLimitDamping=joint_limit_damping
  Hip Roll Joint : walkingRobotUtils/Leg Joint with Limits  VariantControl=actuatorType == 2  k=joint_stiffness  d=joint_damping  initAngle=init_angs_R(4)  eqAngle=0  upperLimit=pi/16  lowerLimit=0  jointLimitStiffness=joint_limit_stiffness  jointLimitDamping=joint_limit_damping
  Hip to World Coords : sm_lib/Frames and Transforms/Rigid Transform  TranslationMethod=None  TranslationStandardOffset=0  TranslationLengthUnit=cm  TranslationStandardAxis=+Z  TranslationCartesianOffset=[0 0 upper_leg_length/2]  TranslationROffset=0  TranslationROffsetUnits=m  TranslationZOffset=0  TranslationZOffsetUnits=m  TranslationThetaOffset=0  TranslationThetaOffsetUnits=deg  RotationMethod=StandardAxis  RotationAngleUnits=deg  RotationStandardAxis=+X  RotationAngle=-90  RotationArbitraryAxis=[0 0 1]  FollAlignAxisA=+X  BaseAlignAxisA=+Y  FollAlignAxisB=+Y  BaseAlignAxisB=+Z  RotationSequenceAxes=FollowerAxes  RotationSequence=XYX  RotationSequenceAngles=[0 0 0]  RotationSequenceAnglesUnits=deg  RotationMatrix=[1 0 0; 0 1 0; 0 0 1]
  Knee Joint : walkingRobotUtils/Leg Joint with Limits  VariantControl=actuatorType == 2  k=joint_stiffness  d=joint_damping  initAngle=init_angs_R(3)  eqAngle=0  upperLimit=pi/2  lowerLimit=0  jointLimitStiffness=joint_limit_stiffness  jointLimitDamping=joint_limit_damping
  Knee to Upper Leg : sm_lib/Frames and Transforms/Rigid Transform  TranslationMethod=Cartesian  TranslationStandardOffset=0  TranslationLengthUnit=cm  TranslationStandardAxis=+Z  TranslationCartesianOffset=[0 upper_leg_length/2 0]  TranslationROffset=0  TranslationROffsetUnits=m  TranslationZOffset=0  TranslationZOffsetUnits=m  TranslationThetaOffset=0  TranslationThetaOffsetUnits=deg  RotationMethod=StandardAxis  RotationAngleUnits=deg  RotationStandardAxis=+X  RotationAngle=-90  RotationArbitraryAxis=[0 0 1]  FollAlignAxisA=+X  BaseAlignAxisA=+Y  FollAlignAxisB=+Y  BaseAlignAxisB=+Z  RotationSequenceAxes=FollowerAxes  RotationSequence=XYX  RotationSequenceAngles=[0 0 0]  RotationSequenceAnglesUnits=deg  RotationMatrix=[1 0 0; 0 1 0; 0 0 1]
  Lower Leg : sm_lib/Body Elements/Cylindrical Solid  GraphicAmbientColor=[0.15 0.15 0.15 1.0]  BasedOnType=Density  CenterOfMass=[0 0 0]  CenterOfMassUnits=m  GraphicDiffuseColor=[0.0 0.8 0.0]  CylinderLength=lower_leg_length  CylinderLengthUnits=cm  CylinderRadius=leg_radius  CylinderRadiusUnits=cm  Density=density  DensityUnits=kg/m^3  DoExposeReferenceFrame=on  GraphicEmissiveColor=[0.0 0.0 0.0 1.0]  ExportEntireGeometry=off  SerializedFrames=<Frames/>  MarkerShape=Sphere  MarkerSize=10  GraphicType=FromGeometry  InertiaType=CalculateFromGeometry  Mass=1  MassUnits=kg  MomentsOfInertia=[1 1 1]  MomentsOfInertiaUnits=kg*m^2  GraphicOpacity=1.0  ProductsOfInertia=[1 1 1]  ProductsOfInertiaUnits=kg*m^2  GraphicShininess=75  GraphicSpecularColor=[0.5 0.5 0.5 1.0]  GraphicVisPropType=SimpleVisualProperties
  Lower Leg to Knee : sm_lib/Frames and Transforms/Rigid Transform  TranslationMethod=Cartesian  TranslationStandardOffset=0  TranslationLengthUnit=cm  TranslationStandardAxis=+Z  TranslationCartesianOffset=[0 0 lower_leg_length/2]  TranslationROffset=0  TranslationROffsetUnits=m  TranslationZOffset=0  TranslationZOffsetUnits=m  TranslationThetaOffset=0  TranslationThetaOffsetUnits=deg  RotationMethod=StandardAxis  RotationAngleUnits=deg  RotationStandardAxis=+X  RotationAngle=90  RotationArbitraryAxis=[0 0 1]  FollAlignAxisA=+X  BaseAlignAxisA=+Y  FollAlignAxisB=+Y  BaseAlignAxisB=+Z  RotationSequenceAxes=FollowerAxes  RotationSequence=XYX  RotationSequenceAngles=[0 0 0]  RotationSequenceAnglesUnits=deg  RotationMatrix=[1 0 0; 0 1 0; 0 0 1]
  Package Measurements 3D : walkingRobotUtils/Package Measurements 3D  SystemSampleTime=-1  VariantActivationTime=update diagram  Latency=0  AutoFrameSizeCalculation=off
  Upper Leg : sm_lib/Body Elements/Cylindrical Solid  GraphicAmbientColor=[0.15 0.15 0.15 1.0]  BasedOnType=Density  CenterOfMass=[0 0 0]  CenterOfMassUnits=m  GraphicDiffuseColor=[0.0 0.0 1.0]  CylinderLength=upper_leg_length  CylinderLengthUnits=cm  CylinderRadius=leg_radius  CylinderRadiusUnits=cm  Density=density  DensityUnits=kg/m^3  DoExposeReferenceFrame=on  GraphicEmissiveColor=[0.0 0.0 0.0 1.0]  ExportEntireGeometry=off  SerializedFrames=<Frames/>  MarkerShape=Sphere  MarkerSize=10  GraphicType=FromGeometry  InertiaType=CalculateFromGeometry  Mass=1  MassUnits=kg  MomentsOfInertia=[1 1 1]  MomentsOfInertiaUnits=kg*m^2  GraphicOpacity=1.0  ProductsOfInertia=[1 1 1]  ProductsOfInertiaUnits=kg*m^2  GraphicShininess=75  GraphicSpecularColor=[0.5 0.5 0.5 1.0]  GraphicVisPropType=SimpleVisualProperties
  Upper Leg to Hip : sm_lib/Frames and Transforms/Rigid Transform  TranslationMethod=Cartesian  TranslationStandardOffset=0  TranslationLengthUnit=cm  TranslationStandardAxis=+Z  TranslationCartesianOffset=[0 0 upper_leg_length/2]  TranslationROffset=0  TranslationROffsetUnits=m  TranslationZOffset=0  TranslationZOffsetUnits=m  TranslationThetaOffset=0  TranslationThetaOffsetUnits=deg  RotationMethod=StandardAxis  RotationAngleUnits=deg  RotationStandardAxis=+X  RotationAngle=90  RotationArbitraryAxis=[0 0 1]  FollAlignAxisA=+X  BaseAlignAxisA=+Y  FollAlignAxisB=+Y  BaseAlignAxisB=+Z  RotationSequenceAxes=FollowerAxes  RotationSequence=XYX  RotationSequenceAngles=[0 0 0]  RotationSequenceAnglesUnits=deg  RotationMatrix=[1 0 0; 0 1 0; 0 0 1]
  G : PMIOPort  Side=Right
  H : PMIOPort  Port=2  Side=Right
  meas : Outport  VectorParamsAs1DForOutWhenUnconnected=off
  wires:
  Knee Joint/1 -> Package Measurements 3D/5
  Hip Pitch Joint/1 -> Package Measurements 3D/7
  Package Measurements 3D/1 -> meas/1
  Ankle Pitch Joint/1 -> Package Measurements 3D/4
  torques/1 -> Demux/1
  Demux/1 -> Ankle Roll Joint/1
  Demux/2 -> Ankle Pitch Joint/1
  Demux/3 -> Knee Joint/1
  Demux/4 -> Hip Roll Joint/1
  Demux/5 -> Hip Pitch Joint/1
  Hip Roll Joint/1 -> Package Measurements 3D/6
  Ankle Roll Joint/1 -> Package Measurements 3D/3
  Foot and Contact/2 -> Package Measurements 3D/2
  Foot and Contact/1 -> Package Measurements 3D/1
  connections:
  H/RConn1 -- Hip to World Coords/RConn1
  Knee Joint/LConn1 -- Lower Leg to Knee/RConn1
  Knee to Upper Leg/RConn1 -- Upper Leg/RConn1 -- Upper Leg to Hip/LConn1
  Lower Leg to Knee/LConn1 -- Lower Leg/RConn1 -- Ankle to Lower Leg/RConn1
  Knee Joint/RConn1 -- Knee to Upper Leg/LConn1
  Ankle Roll Joint/LConn1 -- Ankle Pitch to Roll/RConn1
  Ankle Roll Joint/RConn1 -- Ankle Roll to Pitch/LConn1
  Ankle Pitch Joint/RConn1 -- Ankle to Lower Leg/LConn1
  Hip Pitch Joint/RConn1 -- Hip to World Coords/LConn1
  Hip Roll Joint/LConn1 -- Hip Pitch to Roll/RConn1
  Hip Roll Joint/RConn1 -- Hip Roll to Pitch/LConn1
  Foot Offset/RConn1 -- Ankle Pitch to Roll/LConn1
  Ankle Pitch Joint/LConn1 -- Ankle Roll to Pitch/RConn1
  Upper Leg to Hip/RConn1 -- Hip Pitch to Roll/LConn1
  Hip Roll to Pitch/RConn1 -- Hip Pitch Joint/LConn1
  Foot and Contact/RConn1 -- Foot Offset/LConn1
  G/RConn1 -- Foot and Contact/LConn1

== system walkingRobotRL3D/Walking Robot/Sensors ==
  measR : Inport
  measL : Inport  Port=2
  Add3 : Sum
  Bus Creator : BusCreator  Inputs=18
  Calculate Actuator Power 3D : Subsystem
  Calculate Actuator Power 3D1 : Subsystem
  Demux : Demux  Outputs=3
  Integrator : Integrator
  PS-Simulink Converter{1..9,13..16} (13 alike) : nesl_utility/PS-Simulink Converter  PhysicalDomain=network_engine_domain  SubClassName=ps_output  LeftPortType=input  RightPortType=output  PseudoPeriodic=off  Frequencies=[]  Unit=1  AffineConversion=off
  Rotation Matrix to Roll Pitch Yaw : walkingRobotUtils/Rotation Matrix to  Roll Pitch Yaw  SystemSampleTime=-1  VariantActivationTime=update diagram  Latency=0  AutoFrameSizeCalculation=off
  Transform Sensor : sm_lib/Frames and Transforms/Transform Sensor  MeasurementFrame=World  SenseAngle=off  SenseAxis=off  SenseAngle1=off  SenseAngle2=off  SenseAngle3=off  SenseQ=off  SenseR=on  SenseOmegaX=off  SenseOmegaY=off  SenseOmegaZ=off  SenseOmega1=off  SenseOmega2=off  SenseOmega3=off  SenseQDot=off  SenseRDot=off  SenseAlphaX=off  SenseAlphaY=off  SenseAlphaZ=off  SenseAlpha1=off  SenseAlpha2=off  SenseAlpha3=off  SenseQDDot=off  SenseRDDot=off  SenseX=on  SenseY=on  SenseZ=on  SenseRad=off  SenseAzim=off  SenseDist=off  SenseInc=off  SenseXDot=on  SenseYDot=on  SenseZDot=on  SenseRadDot=off  SenseAzimDot=off  SenseDistDot=off  SenseIncDot=off  SenseXDDot=on  SenseYDDot=on  SenseZDDot=on  SenseRadDDot=off  SenseAzimDDot=off  SenseDistDDot=off  SenseIncDDot=off
  Transform Sensor1 : sm_lib/Frames and Transforms/Transform Sensor  MeasurementFrame=NonRotatingFollower  SenseAngle=off  SenseAxis=off  SenseAngle1=off  SenseAngle2=off  SenseAngle3=off  SenseQ=off  SenseR=off  SenseOmegaX=on  SenseOmegaY=on  SenseOmegaZ=on  SenseOmega1=off  SenseOmega2=off  SenseOmega3=off  SenseQDot=off  SenseRDot=off  SenseAlphaX=off  SenseAlphaY=off  SenseAlphaZ=off  SenseAlpha1=off  SenseAlpha2=off  SenseAlpha3=off  SenseQDDot=off  SenseRDDot=off  SenseX=off  SenseY=off  SenseZ=off  SenseRad=off  SenseAzim=off  SenseDist=off  SenseInc=off  SenseXDot=off  SenseYDot=off  SenseZDot=off  SenseRadDot=off  SenseAzimDot=off  SenseDistDot=off  SenseIncDot=off  SenseXDDot=off  SenseYDDot=off  SenseZDDot=off  SenseRadDDot=off  SenseAzimDDot=off  SenseDistDDot=off  SenseIncDDot=off
  F : PMIOPort  Side=Right
  B : PMIOPort  Port=2  Side=Left
  sensors : Outport  VectorParamsAs1DForOutWhenUnconnected=off
  wires:
  Calculate Actuator Power 3D/1(P) -> Add3/1
  Calculate Actuator Power 3D1/1(P) -> Add3/2
  Add3/1 -> Integrator/1
  Integrator/1 -> Bus Creator/18  "actPower"
  measL/1 -> Calculate Actuator Power 3D1/1(meas), Bus Creator/17  "measL"
  PS-Simulink Converter14/1 -> Bus Creator/13  "wx"
  PS-Simulink Converter15/1 -> Bus Creator/14  "wy"
  Demux/3 -> Bus Creator/3  "roll"
  Bus Creator/1 -> sensors/1
  PS-Simulink Converter9/1 -> Bus Creator/12  "AZ"
  PS-Simulink Converter7/1 -> Bus Creator/7  "VX"
  PS-Simulink Converter8/1 -> Bus Creator/8  "VY"
  Demux/2 -> Bus Creator/2  "pitch"
  PS-Simulink Converter13/1 -> Bus Creator/9  "VZ"
  PS-Simulink Converter4/1 -> Bus Creator/6  "Z"
  Demux/1 -> Bus Creator/1  "yaw"
  measR/1 -> Calculate Actuator Power 3D/1(meas), Bus Creator/16  "measR"
  PS-Simulink Converter5/1 -> Bus Creator/10  "AX"
  PS-Simulink Converter6/1 -> Bus Creator/11  "AY"
  Rotation Matrix to Roll Pitch Yaw/1 -> Demux/1
  PS-Simulink Converter1/1 -> Bus Creator/4  "X"
  PS-Simulink Converter16/1 -> Bus Creator/15  "wz"
  PS-Simulink Converter2/1 -> Bus Creator/5  "Y"
  PS-Simulink Converter3/1 -> Rotation Matrix to Roll Pitch Yaw/1  "R"
  connections:
  F/RConn1 -- Transform Sensor/RConn1 -- Transform Sensor1/RConn1
  B/RConn1 -- Transform Sensor/LConn1 -- Transform Sensor1/LConn1
  PS-Simulink Converter13/LConn1 -- Transform Sensor/RConn8
  Transform Sensor/RConn10 -- PS-Simulink Converter6/LConn1
  Transform Sensor/RConn4 -- PS-Simulink Converter2/LConn1
  Transform Sensor/RConn5 -- PS-Simulink Converter4/LConn1
  Transform Sensor1/RConn4 -- PS-Simulink Converter16/LConn1
  Transform Sensor/RConn7 -- PS-Simulink Converter8/LConn1
  PS-Simulink Converter9/LConn1 -- Transform Sensor/RConn11
  PS-Simulink Converter14/LConn1 -- Transform Sensor1/RConn2
  PS-Simulink Converter1/LConn1 -- Transform Sensor/RConn3
  PS-Simulink Converter15/LConn1 -- Transform Sensor1/RConn3
  PS-Simulink Converter5/LConn1 -- Transform Sensor/RConn9
  PS-Simulink Converter3/LConn1 -- Transform Sensor/RConn2
  PS-Simulink Converter7/LConn1 -- Transform Sensor/RConn6

== system walkingRobotRL3D/Walking Robot/World and Ground ==
  Mechanism Configuration : sm_lib/Utilities/Mechanism Configuration  UniformGravity=Constant  GravityVector=[0 0 -9.80665]  GravityVectorUnits=m/s^2  GravityUnits=m/s^2  LinearizationDelta=0.001  JointModeTransitionNonlinearIterations=2
  Plane Offset : sm_lib/Frames and Transforms/Rigid Transform  TranslationMethod=StandardAxis  TranslationStandardOffset=height_plane/2  TranslationLengthUnit=m  TranslationStandardAxis=-Z  TranslationCartesianOffset=[0 0 0]  TranslationROffset=0  TranslationROffsetUnits=m  TranslationZOffset=0  TranslationZOffsetUnits=m  TranslationThetaOffset=0  TranslationThetaOffsetUnits=deg  RotationMethod=None  RotationAngleUnits=deg  RotationStandardAxis=+Z  RotationAngle=0.0  RotationArbitraryAxis=[0 0 1]  FollAlignAxisA=+X  BaseAlignAxisA=+Y  FollAlignAxisB=+Y  BaseAlignAxisB=+Z  RotationSequenceAxes=FollowerAxes  RotationSequence=XYX  RotationSequenceAngles=[0 0 0]  RotationSequenceAnglesUnits=deg  RotationMatrix=[1 0 0; 0 1 0; 0 0 1]
  Solver Configuration : nesl_utility/Solver Configuration  PhysicalDomain=network_engine_domain  SubClassName=solver  LeftPortType=input  RightPortType=generic  Tones=[]  Harmonics=[]  SimulateNoise=off  Profile=off  UseLocalSampling=off  EnableSwitchedLinearOptims=on  FrequencyDomain=off  UseCCode=off  RelTol=0.001  AbsTol=1e-06  MinStep=1e-09  ToWorkspace=off  RevertToSquareIcSolve=off  NumHomotopyIterations=100  PhasorMode=off  PhasorModeNumHarmonics=1  DoDC=off  ResidualTolerance=1e-09  UseLocalSolver=off  LocalSolverChoice=NE_TRAPEZOIDAL_ADVANCER  LocalSolverSampleTime=Ts  DoFixedCost=off  MaxNonlinIter=3  MaxModeIter=2  ComputeImpulses=off  ImpulseIterations=2  LinearAlgebra=Sparse  EquationFormulation=NE_TIME_EF  DelaysMemoryBudget=1024  AutomaticFiltering=on  FilteringTimeConstant=0.001  PartitionStorageMethod=AS_NEEDED  PartitionMemoryBudget=1024  PartitionMethod=FAST
  World Frame1 : sm_lib/Frames and Transforms/World Frame
  World Plane : sm_lib/Body Elements/Brick Solid  GraphicAmbientColor=[0.15 0.15 0.15 1.0]  BasedOnType=Density  BrickDimensions="[plane_x+10 plane_y  height_plane]"  BrickDimensionUnits=m  CenterOfMass=[0 0 0]  CenterOfMassUnits=m  GraphicDiffuseColor=[1.0 1.0 0.8]  Density=density  DensityUnits=kg/(m^3)  DoExposeReferenceFrame=on  GraphicEmissiveColor=[0.0 0.0 0.0 1.0]  ExportEntireGeometry=on  SerializedFrames=<Frames/>  MarkerShape=Sphere  MarkerSize=10  GraphicType=FromGeometry  InertiaType=CalculateFromGeometry  Mass=1  MassUnits=kg  MomentsOfInertia=[1 1 1]  MomentsOfInertiaUnits=kg*m^2  GraphicOpacity=0.5  ProductsOfInertia=[0 0 0]  ProductsOfInertiaUnits=kg*m^2  GraphicShininess=75  GraphicSpecularColor=[0.5 0.5 0.5 1.0]  GraphicVisPropType=SimpleVisualProperties
  W : PMIOPort  Side=Left
  G : PMIOPort  Port=2  Side=Right
  connections:
  World Frame1/RConn1 -- W/RConn1 -- Mechanism Configuration/RConn1 -- Plane Offset/LConn1 -- Solver Configuration/RConn1
  World Plane/RConn1 -- Plane Offset/RConn1
  G/RConn1 -- World Plane/LConn1

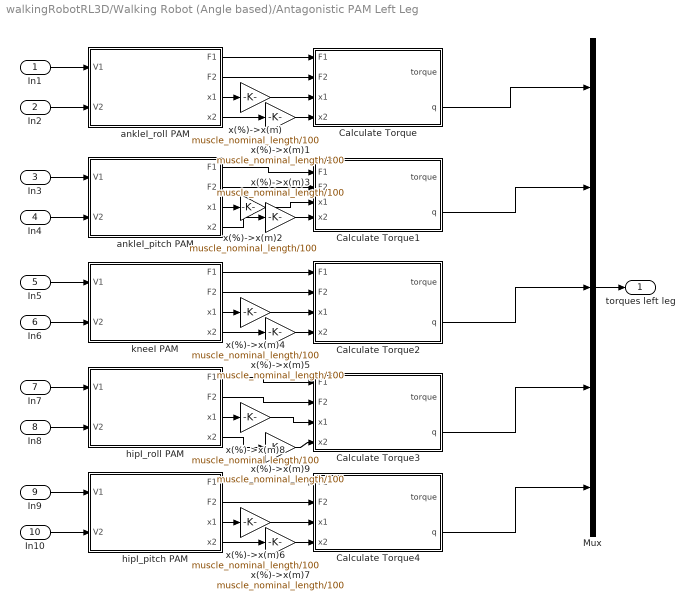
== system walkingRobotRL3D/Walking Robot (Angle based)/Antagonistic PAM Left Leg ==
  In1 : Inport
  In2 : Inport  Port=2
  In3 : Inport  Port=3
  In4 : Inport  Port=4
  In5 : Inport  Port=5
  In6 : Inport  Port=6
  In7 : Inport  Port=7
  In8 : Inport  Port=8
  In9 : Inport  Port=9
  In10 : Inport  Port=10
  Calculate Torque : MATLAB Function  TreatAsAtomicUnit=on
  Calculate Torque1 : MATLAB Function  TreatAsAtomicUnit=on
  Calculate Torque2 : MATLAB Function  TreatAsAtomicUnit=on
  Calculate Torque3 : MATLAB Function  TreatAsAtomicUnit=on
  Calculate Torque4 : MATLAB Function  TreatAsAtomicUnit=on
  Mux : Mux  Inputs=5
  ankleI_pitch PAM : Subsystem
  ankleI_roll PAM : Subsystem
  hipI_pitch PAM : Subsystem
  hipI_roll PAM : Subsystem
  kneeI PAM : Subsystem
  x(%)->x(m){,1..9} (10 alike) : Gain  Gain=muscle_nominal_length/100
  torques left leg : Outport
  wires:
  Mux/1 -> torques left leg/1
  ankleI_roll PAM/1(F1) -> Calculate Torque/1(F1)
  ankleI_roll PAM/2(F2) -> Calculate Torque/2(F2)
  ankleI_roll PAM/3(x1) -> x(%)->x(m)/1
  ankleI_roll PAM/4(x2) -> x(%)->x(m)1/1
  ankleI_pitch PAM/1(F1) -> Calculate Torque1/1(F1)
  ankleI_pitch PAM/2(F2) -> Calculate Torque1/2(F2)
  kneeI PAM/1(F1) -> Calculate Torque2/1(F1)
  kneeI PAM/2(F2) -> Calculate Torque2/2(F2)
  kneeI PAM/3(x1) -> x(%)->x(m)4/1
  kneeI PAM/4(x2) -> x(%)->x(m)5/1
  hipI_roll PAM/1(F1) -> Calculate Torque3/1(F1)
  hipI_roll PAM/2(F2) -> Calculate Torque3/2(F2)
  hipI_pitch PAM/1(F1) -> Calculate Torque4/1(F1)
  hipI_pitch PAM/2(F2) -> Calculate Torque4/2(F2)
  hipI_pitch PAM/3(x1) -> x(%)->x(m)6/1
  hipI_pitch PAM/4(x2) -> x(%)->x(m)7/1
  Calculate Torque/2(q) -> Mux/1
  Calculate Torque1/2(q) -> Mux/2
  Calculate Torque2/2(q) -> Mux/3
  Calculate Torque3/2(q) -> Mux/4
  Calculate Torque4/2(q) -> Mux/5
  x(%)->x(m)/1 -> Calculate Torque/3(x1)
  x(%)->x(m)1/1 -> Calculate Torque/4(x2)
  x(%)->x(m)2/1 -> Calculate Torque1/3(x1)
  ankleI_pitch PAM/3(x1) -> x(%)->x(m)2/1
  x(%)->x(m)3/1 -> Calculate Torque1/4(x2)
  ankleI_pitch PAM/4(x2) -> x(%)->x(m)3/1
  x(%)->x(m)4/1 -> Calculate Torque2/3(x1)
  x(%)->x(m)5/1 -> Calculate Torque2/4(x2)
  x(%)->x(m)6/1 -> Calculate Torque4/3(x1)
  x(%)->x(m)7/1 -> Calculate Torque4/4(x2)
  hipI_roll PAM/3(x1) -> x(%)->x(m)8/1
  x(%)->x(m)8/1 -> Calculate Torque3/3(x1)
  x(%)->x(m)9/1 -> Calculate Torque3/4(x2)
  hipI_roll PAM/4(x2) -> x(%)->x(m)9/1
  In1/1 -> ankleI_roll PAM/1(V1)
  In2/1 -> ankleI_roll PAM/2(V2)
  In3/1 -> ankleI_pitch PAM/1(V1)
  In4/1 -> ankleI_pitch PAM/2(V2)
  In5/1 -> kneeI PAM/1(V1)
  In6/1 -> kneeI PAM/2(V2)
  In7/1 -> hipI_roll PAM/1(V1)
  In8/1 -> hipI_roll PAM/2(V2)
  In9/1 -> hipI_pitch PAM/1(V1)
  In10/1 -> hipI_pitch PAM/2(V2)
